simulink subsystem "MagField_mea_sim"  (R2024a)
settings: Solver=VariableStepAuto  StartTime=0.0  StopTime=10.0  RelTol=1e-3
undefined symbols (not defined in the file or in its folder): WMM2020
libraries: aerolibutil x1, aerolibgravity2 x1
settings Model: Creator=ruimi  LastModifiedBy=ruimi

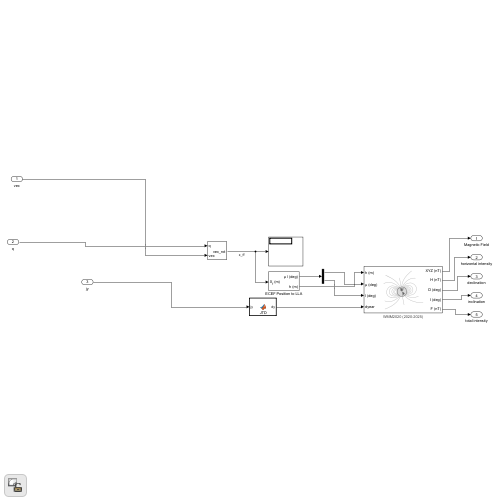
[thumbnail: Simulink's stored preview of the top-level diagram]
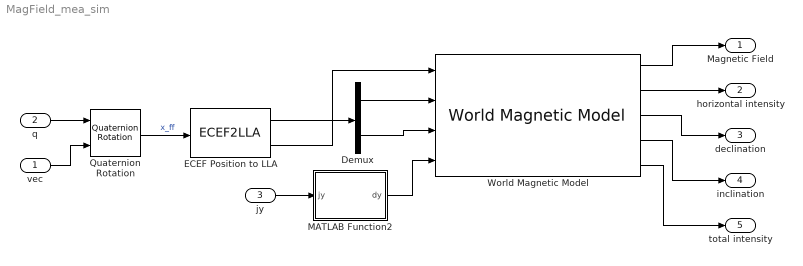
== system MagField_mea_sim ==
  vec : Inport
  q : Inport  Port=2
  jy : Inport  Port=3
  Demux : Demux  Outputs=2
  ECEF Position to LLA : ECEF2LLA
  MATLAB Function2 : MATLAB Function  TreatAsAtomicUnit=on
  Quaternion Rotation : aerolibutil/Quaternion Rotation
  World Magnetic Model : aerolibgravity2/World Magnetic Model  model=WMM2020 (2020-2025)  customFile='WMM2020.COF'  units=Metric (MKS)  time_in=on  month=January  day=1  year=2020  action=None  h_out=on  dec_out=on  inc_out=on  ti_out=on
  Magnetic Field : Outport
  horizontal intensity : Outport  Port=2
  declination : Outport  Port=3
  inclination : Outport  Port=4
  total intensity : Outport  Port=5
  wires:
  vec/1 -> Quaternion Rotation/2
  Demux/2 -> World Magnetic Model/3
  Demux/1 -> World Magnetic Model/2
  jy/1 -> MATLAB Function2/1(jy)
  q/1 -> Quaternion Rotation/1
  Quaternion Rotation/1 -> ECEF Position to LLA/1  "x_ff"
  ECEF Position to LLA/2 -> World Magnetic Model/1
  ECEF Position to LLA/1 -> Demux/1
  MATLAB Function2/1(dy) -> World Magnetic Model/4
  World Magnetic Model/1 -> Magnetic Field/1
  World Magnetic Model/2 -> horizontal intensity/1
  World Magnetic Model/3 -> declination/1
  World Magnetic Model/4 -> inclination/1
  World Magnetic Model/5 -> total intensity/1

== matlab function MagField_mea_sim/MATLAB Function2 ==
  data: jy input; dy output
function dy= JTD(jy)
    %disp('enter JTD_mea')
    dy = JulianToDecimal(jy);
end
